simulink model "prob4"  (R2020b)
settings: Solver=VariableStepAuto  StartTime=0.0  StopTime=10.0  RelTol=1e-3
libraries: dspsrcs4 x1
settings Model: Creator=DELL  LastModifiedBy=DELL

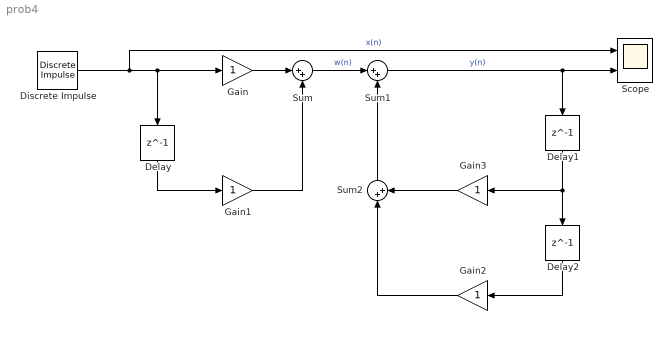
== system prob4 ==
  Delay : Delay  DelayLength=1
  Delay1 : Delay  DelayLength=1
  Delay2 : Delay  DelayLength=1
  Discrete Impulse : dspsrcs4/Discrete  Impulse  Delay=0  SampleTime=1  FrameSample=1  OutputFrames=off  dataType=double  isSigned=on  wordLen=16  udDataType=sfix(16)  fracBitsMode=Best precision  numFracBits=15  OutDataTypeStr=double  LastOutDataTypeStr=double
  Gain{,1..3} (4 alike) : Gain
  Scope : Scope  NumInputPorts=2
  Sum : Sum  Inputs=|++
  Sum1 : Sum  Inputs=|++
  Sum2 : Sum  Inputs=|++
  wires:
  Discrete Impulse/1 -> Scope/1, Delay/1, Gain/1  "x(n)"
  Delay/1 -> Gain1/1
  Gain/1 -> Sum/1
  Gain1/1 -> Sum/2
  Sum/1 -> Sum1/1  "w(n)"
  Sum2/1 -> Sum1/2
  Gain3/1 -> Sum2/2
  Delay1/1 -> Delay2/1, Gain3/1
  Delay2/1 -> Gain2/1
  Gain2/1 -> Sum2/1
  Sum1/1 -> Scope/2, Delay1/1  "y(n)"
